simulink model "KalmanClean"  (R2018a)
settings: Solver=ode4  StartTime=0.0  StopTime=10.0  FixedStep=0.01  RelTol=1e-3
values from neighbouring files (symbols this model uses):
  A = [1 0;     k/m b/m]    [Kalman.m]    (also in fcn.m = [0 1;     -k/m -b/m]; temtProp.m = [0 1;-g/l 0]; untitled2.m = [0 1;     -k/m -b/m])
  B = [0; 1]    [Kalman.m]    (also in fcn.m = [0; 1/m]; temtProp.m = [0;1/(m*l^2)]; untitled2.m = [0; 1/m])
  C = [1 0]    [Kalman.m]    (also in fcn.m = [0 1]; temtProp.m; untitled2.m = [0 1])
  p_pri = A*p_zero*A'    [Kalman.m]    (also in fcn.m = A*p*A + Q)
  R = 1    [Kalman.m]    (also in fcn.m = 0.0001; temtProp.m = 0.0001; untitled2.m = 1-e4)
  x_hzero = [11; 0]    [Kalman.m]    (also in fcn.m = [10; 0]; untitled2.m = [5; 0])
settings Model: Creator=Ali  LastModifiedBy=Ali

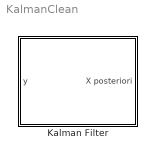
== system KalmanClean ==
  Kalman Filter : Subsystem

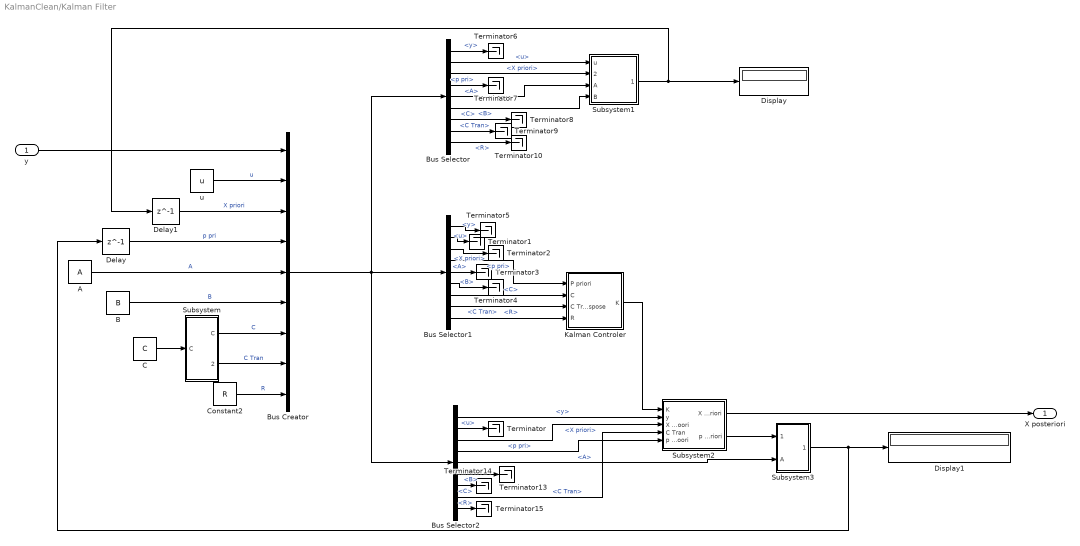
== system KalmanClean/Kalman Filter ==
  y : Inport
  A : Constant  Value=A
  B : Constant  Value=B
  Bus Creator : BusCreator  Inputs=9
  Bus Selector : BusSelector  OutputSignals=y,u,X priori,p pri,A,B,C,C Tran,R
  Bus Selector1 : BusSelector  OutputSignals=y,u,X priori,p pri,A,B,C,C Tran,R
  Bus Selector2 : BusSelector  OutputSignals=y,u,X priori,p pri,A,B,C,C Tran,R
  C : Constant  Value=C
  Constant2 : Constant  Value=R
  Delay : Delay  DelayLength=1  InitialCondition=p_pri
  Delay1 : Delay  DelayLength=1  InitialCondition=x_hzero
  Display : Display
  Display1 : Display
  Kalman Controler : Subsystem
  Subsystem : Subsystem
  Subsystem1 : Subsystem
  Subsystem2 : Subsystem
  Subsystem3 : Subsystem
  Terminator{,1..10,13..15} (14 alike) : Terminator
  u : Constant  Value=u
  X posteriori : Outport
  wires:
  Bus Selector2/5 -> Subsystem3/2(A)  "<A>"
  Kalman Controler/1(K) -> Subsystem2/1(K)
  Bus Selector/4 -> Terminator7/1  "<p pri>"
  Subsystem2/2(p posteriori) -> Subsystem3/1(In1)
  Bus Selector1/3 -> Terminator2/1  "<X priori>"
  Bus Selector1/9 -> Kalman Controler/4(R)  "<R>"
  Bus Selector2/6 -> Terminator13/1  "<B>"
  Bus Selector2/3 -> Subsystem2/3(X prioori)  "<X priori>"
  A/1 -> Bus Creator/5  "A"
  Subsystem2/1(X posteriori) -> X posteriori/1
  Bus Selector1/2 -> Terminator1/1  "<u>"
  Subsystem/2(C Tran) -> Bus Creator/8  "C Tran"
  Bus Selector/9 -> Terminator10/1  "<R>"
  C/1 -> Subsystem/1(C)
  Subsystem/1("C ") -> Bus Creator/7  "C"
  Bus Selector2/8 -> Subsystem2/4(C Tran)  "<C Tran>"
  Bus Selector/1 -> Terminator6/1  "<y>"
  Bus Selector1/1 -> Terminator5/1  "<y>"
  u/1 -> Bus Creator/2  "u"
  Bus Selector/3 -> Subsystem1/2(x hat zero)  "<X priori>"
  Bus Selector1/5 -> Terminator3/1  "<A>"
  Bus Selector2/9 -> Terminator15/1  "<R>"
  Bus Creator/1 -> Bus Selector2/1, Bus Selector1/1, Bus Selector/1
  Delay1/1 -> Bus Creator/3  "X priori"
  B/1 -> Bus Creator/6  "B"
  Bus Selector1/4 -> Kalman Controler/1(P priori)  "<p pri>"
  Bus Selector/6 -> Subsystem1/4(B)  "<B>"
  y/1 -> Bus Creator/1
  Bus Selector2/1 -> Subsystem2/2(y)  "<y>"
  Bus Selector2/7 -> Terminator14/1  "<C>"
  Delay/1 -> Bus Creator/4  "p pri"
  Bus Selector/8 -> Terminator9/1  "<C Tran>"
  Bus Selector2/4 -> Subsystem2/5(p prioori)  "<p pri>"
  Bus Selector2/2 -> Terminator/1  "<u>"
  Bus Selector/5 -> Subsystem1/3(A)  "<A>"
  Bus Selector/7 -> Terminator8/1  "<C>"
  Bus Selector1/8 -> Kalman Controler/3(C Transpose)  "<C Tran>"
  Bus Selector/2 -> Subsystem1/1(u)  "<u>"
  Constant2/1 -> Bus Creator/9  "R"
  Subsystem3/1(P pri) -> Delay/1, Display1/1
  Bus Selector1/7 -> Kalman Controler/2(C)  "<C>"
  Subsystem1/1(X priori) -> Delay1/1, Display/1
  Bus Selector1/6 -> Terminator4/1  "<B>"

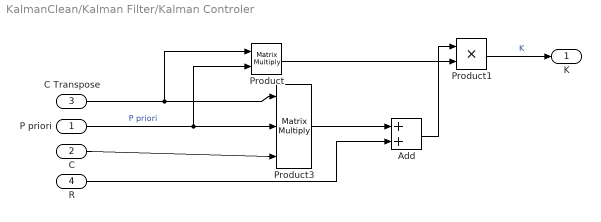
== system KalmanClean/Kalman Filter/Kalman Controler ==
  P priori : Inport
  C : Inport  Port=2
  C Transpose : Inport  Port=3
  R : Inport  Port=4
  Add : Sum
  Product : Product  Multiplication=Matrix(*)
  Product1 : Product
  Product3 : Product  Inputs=3  Multiplication=Matrix(*)
  K : Outport
  wires:
  C/1 -> Product3/3
  R/1 -> Add/2
  Product3/1 -> Add/1
  Add/1 -> Product1/1
  C Transpose/1 -> Product/1, Product3/1
  Product1/1 -> K/1  "K"
  Product/1 -> Product1/2
  P priori/1 -> Product/2, Product3/2  "P priori"

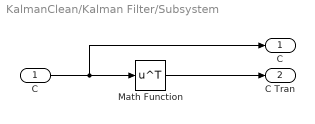
== system KalmanClean/Kalman Filter/Subsystem ==
  C : Inport
  Math Function : Math  Operator=transpose  SaturateOnIntegerOverflow=on
  "C " : Outport
  C Tran : Outport  Port=2
  wires:
  C/1 -> "C "/1, Math Function/1
  Math Function/1 -> C Tran/1

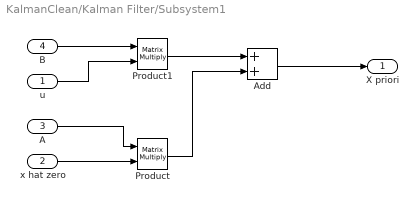
== system KalmanClean/Kalman Filter/Subsystem1 ==
  u : Inport
  x hat zero : Inport  Port=2
  A : Inport  Port=3
  B : Inport  Port=4
  Add : Sum
  Product : Product  Multiplication=Matrix(*)
  Product1 : Product  Multiplication=Matrix(*)
  X priori : Outport
  wires:
  A/1 -> Product/1
  Add/1 -> X priori/1
  u/1 -> Product1/2
  B/1 -> Product1/1
  x hat zero/1 -> Product/2
  Product1/1 -> Add/1
  Product/1 -> Add/2

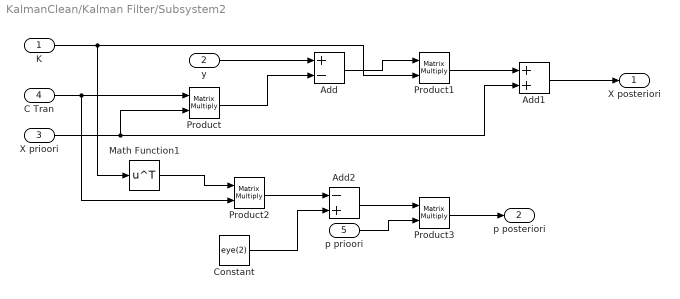
== system KalmanClean/Kalman Filter/Subsystem2 ==
  K : Inport
  y : Inport  Port=2
  X prioori : Inport  Port=3
  C Tran : Inport  Port=4
  p prioori : Inport  Port=5
  Add : Sum  Inputs=+-
  Add1 : Sum
  Add2 : Sum  Inputs=-+
  Constant : Constant  Value=eye(2)
  Math Function1 : Math  Operator=transpose  SaturateOnIntegerOverflow=on
  Product{,1..3} (4 alike) : Product  Multiplication=Matrix(*)
  X posteriori : Outport
  p posteriori : Outport  Port=2
  wires:
  Add1/1 -> X posteriori/1
  Add/1 -> Product1/1
  y/1 -> Add/1
  Product/1 -> Add/2
  Product1/1 -> Add1/1
  X prioori/1 -> Add1/2, Product/2
  Product2/1 -> Add2/1
  Constant/1 -> Add2/2
  K/1 -> Math Function1/1, Product1/2
  C Tran/1 -> Product2/2, Product/1
  Math Function1/1 -> Product2/1
  p prioori/1 -> Product3/2
  Add2/1 -> Product3/1
  Product3/1 -> p posteriori/1

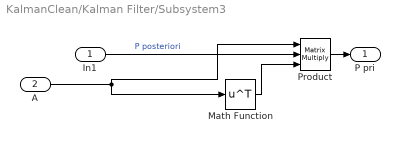
== system KalmanClean/Kalman Filter/Subsystem3 ==
  In1 : Inport
  A : Inport  Port=2
  Math Function : Math  Operator=transpose  SaturateOnIntegerOverflow=on
  Product : Product  Inputs=3  Multiplication=Matrix(*)
  P pri : Outport
  wires:
  Product/1 -> P pri/1
  A/1 -> Product/1, Math Function/1
  In1/1 -> Product/2  "P posteriori"
  Math Function/1 -> Product/3
